simulink model "test_direct"  (R2024a)
settings: Solver=VariableStepAuto  StartTime=0.0  StopTime=40  RelTol=1e-3
libraries: neural x733, simulink x4
(part 20 of 35)

== system test_direct/Function Fitting Neural Network3/Layer 4/Delays 1 ==
  "p{4}" : Inport  PortDimensions=20
      mask Display: e = 0.06;c1 = [120 230 180]/255;c2 = ([120 230 180]+0)/(256+128);c3 = ([120 230 180]+128)/(256+128);patch([0 1 1 0],[0 0 1 1],c1);patch([0 1 1 1-e 1-e 0+e],[0 0 1 1-e 0+e 0+e],c2);patch([0 0 1 1-e 0+e 0+e],[0 1 1 1-e 1-e 0+e],c3);plot([0 1 1 0 0],[0 0 1 1 0]);
  mux : Mux  Inputs=1
      mask Display: e = 0.06;c1 = [120 150 230]/255;c2 = ([120 150 230]+0)/383;c3 = ([120 150 230]+128)/383;patch([0 1 1 0],[0 0 1 1],c1);patch([0 1 1 1-e 1-e 0+e],[0 0 1 1-e 0+e 0+e],c2);patch([0 0 1 1-e 0+e 0+e],[0 1 1 1-e 1-e 0+e],c3);plot([0 1 1 0 0],[0 0 1 1 0]);disp('Mux')
  "pd{4,3}" : Outport
      mask Display: e = 0.06;c1 = [120 230 180]/255;c2 = ([120 230 180]+0)/(256+128);c3 = ([120 230 180]+128)/(256+128);patch([0 1 1 0],[0 0 1 1],c1);patch([0 1 1 1-e 1-e 0+e],[0 0 1 1-e 0+e 0+e],c2);patch([0 0 1 1-e 0+e 0+e],[0 1 1 1-e 1-e 0+e],c3);plot([0 1 1 0 0],[0 0 1 1 0]);
  wires:
  "p{4}"/1 -> mux/1
  mux/1 -> "pd{4,3}"/1

== system test_direct/Function Fitting Neural Network3/Layer 4/LW{4,3} ==
  "ad{4,3}" : Inport  PortDimensions=20
      mask Display: e = 0.06;c1 = [120 230 180]/255;c2 = ([120 230 180]+0)/(256+128);c3 = ([120 230 180]+128)/(256+128);patch([0 1 1 0],[0 0 1 1],c1);patch([0 1 1 1-e 1-e 0+e],[0 0 1 1-e 0+e 0+e],c2);patch([0 0 1 1-e 0+e 0+e],[0 1 1 1-e 1-e 0+e],c3);plot([0 1 1 0 0],[0 0 1 1 0]);
  "IW{4,3}(1,:)'" : Constant  Value=[-0.48686646195795912905879276877385564148426055908203125;-0.039175733463625579677813703938227263279259204864501953125;-0.054262605722279790010365019270466291345655918121337890625;-0.0940799827120739617924982667318545281887054443359375;0.368204999001782551371064755585393868386745452880859375;-0.060856578835075413047572823188602342270314693450927734375;-0.016079589379415247518689824346438399516046047210693359375;-0.5573541309042620017777380780898965895175933837890625;-0.410950220679517475019792982493527233600616455078125;-0.456090081196367957971915529924444854259490966796875;-0.086733219532944494378767785747186280786991119384765625;-0.442442468295296709168695770131307654082775115966796875;0.181816513039095795090105411873082630336284637451171875;0.324817807046969997397667384575470350682735443115234375;0.0251481921723479238950371694727436988614499568939208984375;-0.233647632030154317472891989382333122193813323974609375;0.47822246659309808336502101155929267406463623046875;-0.281298981443819762215952096084947697818279266357421875;-0.342982629902267077692812335953931324183940887451171875;0.111229079439892408753820518541033379733562469482421875]
      mask Display: e = 0.06;c1 = [120 150 230]/255;c2 = ([120 150 230]+0)/383;c3 = ([120 150 230]+128)/383;patch([0 1 1 0],[0 0 1 1],c1);patch([0 1 1 1-e 1-e 0+e],[0 0 1 1-e 0+e 0+e],c2);patch([0 0 1 1-e 0+e 0+e],[0 1 1 1-e 1-e 0+e],c3);plot([0 1 1 0 0],[0 0 1 1 0]);disp('weights');
  "IW{4,3}(10,:)'" : Constant  Value=[0.1322689043770106653852280942373909056186676025390625;0.58032543371156875000593799995840527117252349853515625;0.2470434001325927386716330147464759647846221923828125;0.381612023463914373788696821065968833863735198974609375;0.46510415946604710679679328677593730390071868896484375;0.36918358843860288320826157359988428652286529541015625;0.10829240045879288956154340439752559177577495574951171875;0.438447426649319738078958152982522733509540557861328125;-0.475651030999239221586094572558067739009857177734375;0.5174868322376242613103158873855136334896087646484375;0.46252837137097035924426791098085232079029083251953125;0.351788445832689256054237603166257031261920928955078125;0.2169410354624995151961996953104971908032894134521484375;-0.003875396627683679907916403095669011236168444156646728515625;0.04911082881832169733105075692947139032185077667236328125;0.052739315397494108961229386522973072715103626251220703125;-0.05480510469211240243136984418015344999730587005615234375;-0.53198177995099904524778366976534016430377960205078125;-0.10334524086508810325479856828678748570382595062255859375;0.375453827597210965105745117398328147828578948974609375]
      mask Display: e = 0.06;c1 = [120 150 230]/255;c2 = ([120 150 230]+0)/383;c3 = ([120 150 230]+128)/383;patch([0 1 1 0],[0 0 1 1],c1);patch([0 1 1 1-e 1-e 0+e],[0 0 1 1-e 0+e 0+e],c2);patch([0 0 1 1-e 0+e 0+e],[0 1 1 1-e 1-e 0+e],c3);plot([0 1 1 0 0],[0 0 1 1 0]);disp('weights');
  "IW{4,3}(2,:)'" : Constant  Value=[0.394185608854831726066691999221802689135074615478515625;-0.73688134269214800031733147989143617451190948486328125;0.07487875784436172355018612734056659974157810211181640625;0.422127005558921297723173893245984800159931182861328125;-0.1848428640511568799009722852133563719689846038818359375;0.093106201221737350248730535895447246730327606201171875;-0.639864400764405427679548665764741599559783935546875;-0.45328319723072063585078694814001210033893585205078125;0.58552337302374535266125121779623441398143768310546875;0.1926483079783262442052915730528184212744235992431640625;-0.60409923873878768052492205242742784321308135986328125;0.468018274699262659677145848036161623895168304443359375;-0.8511680335689548737576615167199634015560150146484375;0.024315010267243752917210031228023581206798553466796875;0.224700621110978493444321202332503162324428558349609375;-0.0016341048010425356269703645040181072545237839221954345703125;0.020521423701335757272534721096235443837940692901611328125;-0.214964210107415232275940297768102027475833892822265625;0.48652592408502892684651897070580162107944488525390625;-0.50226604360123972004004144764621742069721221923828125]
      mask Display: e = 0.06;c1 = [120 150 230]/255;c2 = ([120 150 230]+0)/383;c3 = ([120 150 230]+128)/383;patch([0 1 1 0],[0 0 1 1],c1);patch([0 1 1 1-e 1-e 0+e],[0 0 1 1-e 0+e 0+e],c2);patch([0 0 1 1-e 0+e 0+e],[0 1 1 1-e 1-e 0+e],c3);plot([0 1 1 0 0],[0 0 1 1 0]);disp('weights');
  "IW{4,3}(3,:)'" : Constant  Value=[-0.2491793519076358764952061619624146260321140289306640625;0.2423952947801428503549203696820768527686595916748046875;-0.446054257266220999245120992782176472246646881103515625;-0.54592514430021055193975598740507848560810089111328125;0.339034794585557353041593842135625891387462615966796875;0.1746683376047669933317507684478187002241611480712890625;-0.352707257123562489820045584565377794206142425537109375;0.045936039691991246980418139855828485451638698577880859375;-0.1638667128451297971825084687225171364843845367431640625;0.250704205658886014607134029574808664619922637939453125;-0.294664529227201210659359276178292930126190185546875;-0.42733283149903389386281560291536152362823486328125;0.2269107231504099153607256766917998902499675750732421875;0.57311441583918953934784212833619676530361175537109375;-0.30882524085834373028802701810491271317005157470703125;0.42145837800391727778759332068148069083690643310546875;0.01697039272420101940763714765125769190490245819091796875;0.33169200899486928069137547936406917870044708251953125;-0.493372721243436063165432869936921633780002593994140625;0.6407201682409671139595275235478766262531280517578125]
      mask Display: e = 0.06;c1 = [120 150 230]/255;c2 = ([120 150 230]+0)/383;c3 = ([120 150 230]+128)/383;patch([0 1 1 0],[0 0 1 1],c1);patch([0 1 1 1-e 1-e 0+e],[0 0 1 1-e 0+e 0+e],c2);patch([0 0 1 1-e 0+e 0+e],[0 1 1 1-e 1-e 0+e],c3);plot([0 1 1 0 0],[0 0 1 1 0]);disp('weights');
  "IW{4,3}(4,:)'" : Constant  Value=[-0.185259915495485427694433155920705758035182952880859375;-0.0602096723483524220998930331916199065744876861572265625;0.005160964867985998703880934357357546105049550533294677734375;-0.28022125227828265092711035322281531989574432373046875;-0.260470767970210126396324312736396677792072296142578125;-0.061202911858095128405654605785457533784210681915283203125;-0.1114271602009062334115441217363695614039897918701171875;0.65705660638789586958097288516000844538211822509765625;0.0274548355082907501178990372636690153740346431732177734375;0.0196237861339672824134705564347314066253602504730224609375;0.181669946716588370794198681323905475437641143798828125;-0.337641594933245914322839098531403578817844390869140625;-0.1374064240998444652586130132476682774722576141357421875;-0.1853221345637752204282833190518431365489959716796875;-0.65902271493018016457199337310157716274261474609375;-0.1235825644534767897564364602658315561711788177490234375;-0.2164996901666107198547450707337702624499797821044921875;0.465730287211794602431069733938784338533878326416015625;-0.0225226151377865453639959270049075712449848651885986328125;0.453007245753051457359816822645370848476886749267578125]
      mask Display: e = 0.06;c1 = [120 150 230]/255;c2 = ([120 150 230]+0)/383;c3 = ([120 150 230]+128)/383;patch([0 1 1 0],[0 0 1 1],c1);patch([0 1 1 1-e 1-e 0+e],[0 0 1 1-e 0+e 0+e],c2);patch([0 0 1 1-e 0+e 0+e],[0 1 1 1-e 1-e 0+e],c3);plot([0 1 1 0 0],[0 0 1 1 0]);disp('weights');
  "IW{4,3}(5,:)'" : Constant  Value=[-0.428439923209114059687863118597306311130523681640625;-0.479089500144313007456986497345496900379657745361328125;-0.475435563334728195084011304061277769505977630615234375;0.28555488193449340972307481933967210352420806884765625;-0.0671512868641155058480052275626803748309612274169921875;-0.103174105025102991195495860665687359869480133056640625;0.1779694070506021574828992015682160854339599609375;-0.4165875142106241213468820205889642238616943359375;0.11253138387435483724896556623207288794219493865966796875;-0.414639990588654028247361793546588160097599029541015625;0.5106068345219061388462478134897537529468536376953125;-0.442561665969515571905645856531918980181217193603515625;0.1283178924385620367498717087073600850999355316162109375;0.288453901604045104267726173929986543953418731689453125;0.4438188348713214548268979342537932097911834716796875;0.31938958024108232702786835943697951734066009521484375;-0.08115556966456148602073739084517001174390316009521484375;0.293674793410225898337984062891337089240550994873046875;0.2448754137198137226238969788028043694794178009033203125;0.5552223354759082685205839879927225410938262939453125]
      mask Display: e = 0.06;c1 = [120 150 230]/255;c2 = ([120 150 230]+0)/383;c3 = ([120 150 230]+128)/383;patch([0 1 1 0],[0 0 1 1],c1);patch([0 1 1 1-e 1-e 0+e],[0 0 1 1-e 0+e 0+e],c2);patch([0 0 1 1-e 0+e 0+e],[0 1 1 1-e 1-e 0+e],c3);plot([0 1 1 0 0],[0 0 1 1 0]);disp('weights');
  "IW{4,3}(6,:)'" : Constant  Value=[-0.49335970568954834458708091915468685328960418701171875;0.627254380166531344542590886703692376613616943359375;-0.42687565884003342286945326122804544866085052490234375;-0.8096754077238739188970839677494950592517852783203125;-0.57129515370796724038626734909485094249248504638671875;0.5820748227951784148359593018540181219577789306640625;0.85048395815353872162489778929739259183406829833984375;0.08899992698425469861422953954388503916561603546142578125;-1.08570552066859793427511249319650232791900634765625;0.462303758497051131559629766343277879059314727783203125;-0.903259753431511658305907985777594149112701416015625;0.10726998787899404141921166910833562724292278289794921875;0.465031374451071066733476300214533694088459014892578125;-0.45929324220655354249487345441593788564205169677734375;-0.56223262128137729831678370828740298748016357421875;0.339090944158511431449909423463395796716213226318359375;-0.11761342441935905556160690821343450807034969329833984375;-0.37686279254677323979905168016557581722736358642578125;0.04121241225336517988164786174820619635283946990966796875;-0.2042736093037561817542524522650637663900852203369140625]
      mask Display: e = 0.06;c1 = [120 150 230]/255;c2 = ([120 150 230]+0)/383;c3 = ([120 150 230]+128)/383;patch([0 1 1 0],[0 0 1 1],c1);patch([0 1 1 1-e 1-e 0+e],[0 0 1 1-e 0+e 0+e],c2);patch([0 0 1 1-e 0+e 0+e],[0 1 1 1-e 1-e 0+e],c3);plot([0 1 1 0 0],[0 0 1 1 0]);disp('weights');
  "IW{4,3}(7,:)'" : Constant  Value=[-0.06537952429101571982794638415725785307586193084716796875;0.0686118153796015095569060804336913861334323883056640625;-0.2105712354158649490809551707570790313184261322021484375;0.05224571883096605640073306631165905855596065521240234375;0.007546513790575325175691290269242017529904842376708984375;0.083163865197247666127822185444529168307781219482421875;0.27287292560545661768145464520785026252269744873046875;0.438194139001469362693086395665886811912059783935546875;-0.034300814531695124343091407581596286036074161529541015625;0.51963615226882031716826304545975290238857269287109375;0.6487591374666166199602912456612102687358856201171875;-0.463435073667250396756145391918835230171680450439453125;0.002905004743866214378389400962987565435469150543212890625;0.73084099932672652588649953031563200056552886962890625;-0.4272768910794726426871648072847165167331695556640625;0.3072026547358976955592879676260054111480712890625;-0.307773827519164100419146734566311351954936981201171875;-0.283230198793040177651647582024452276527881622314453125;-0.1218488722444253935517366471685818396508693695068359375;-0.00267663631928003430127116502035278244875371456146240234375]
      mask Display: e = 0.06;c1 = [120 150 230]/255;c2 = ([120 150 230]+0)/383;c3 = ([120 150 230]+128)/383;patch([0 1 1 0],[0 0 1 1],c1);patch([0 1 1 1-e 1-e 0+e],[0 0 1 1-e 0+e 0+e],c2);patch([0 0 1 1-e 0+e 0+e],[0 1 1 1-e 1-e 0+e],c3);plot([0 1 1 0 0],[0 0 1 1 0]);disp('weights');
  "IW{4,3}(8,:)'" : Constant  Value=[0.5905066251936845755921012823819182813167572021484375;-0.30329863794689615463795462346752174198627471923828125;-0.09760906261871506173211088253083289600908756256103515625;-0.2429638526781317808822535653234808705747127532958984375;0.3234179069280116447515638355980627238750457763671875;-0.42333294766016471566416612404282204806804656982421875;0.3236234153818726699824992465437389910221099853515625;0.441875449522532603996438638205290772020816802978515625;0.5068013555949091308860943172476254403591156005859375;-0.1972272324421973921371176174943684600293636322021484375;0.0480240103525966521846868317879852838814258575439453125;0.444141970587676127024678862653672695159912109375;-0.2197429979112982822986310793567099608480930328369140625;-0.6816575021358606267796176325646229088306427001953125;-0.7021329850213240408862702679471112787723541259765625;-0.411567756854281541212259298845310695469379425048828125;-0.1317867912264614194128853341680951416492462158203125;-0.462287294868110543166750403543119318783283233642578125;0.34924752008150428128629982893471606075763702392578125;0.10496481903143962954860768377329804934561252593994140625]
      mask Display: e = 0.06;c1 = [120 150 230]/255;c2 = ([120 150 230]+0)/383;c3 = ([120 150 230]+128)/383;patch([0 1 1 0],[0 0 1 1],c1);patch([0 1 1 1-e 1-e 0+e],[0 0 1 1-e 0+e 0+e],c2);patch([0 0 1 1-e 0+e 0+e],[0 1 1 1-e 1-e 0+e],c3);plot([0 1 1 0 0],[0 0 1 1 0]);disp('weights');
  "IW{4,3}(9,:)'" : Constant  Value=[0.43056348001155819726903928312822245061397552490234375;0.00111634494525898330004320957442587314289994537830352783203125;-0.528135750842535944826749982894398272037506103515625;-0.307078785122185227152158404351212084293365478515625;-0.03333149626931240783189736021085991524159908294677734375;-0.1371153453742978423068876736579113639891147613525390625;-0.06662096833313123356301588273709057830274105072021484375;0.452089390549744785108288169794832356274127960205078125;0.67958178908102506721178315274300985038280487060546875;-0.362801795077034749947841874018195085227489471435546875;0.339735254339901426856584976121666841208934783935546875;-0.4909941905178099030848670736304484307765960693359375;0.330655951855933827321365470197633840143680572509765625;-0.339969929699753758978175710581126622855663299560546875;-0.0965979905593430110410935185427661053836345672607421875;0.1254839413117765645200307744744350202381610870361328125;0.35972773789546763634206172355334274470806121826171875;-0.2147232346809808678500530731980688869953155517578125;0.48694385960235730959055899802478961646556854248046875;0.172732370055611317294363971086568199098110198974609375]
      mask Display: e = 0.06;c1 = [120 150 230]/255;c2 = ([120 150 230]+0)/383;c3 = ([120 150 230]+128)/383;patch([0 1 1 0],[0 0 1 1],c1);patch([0 1 1 1-e 1-e 0+e],[0 0 1 1-e 0+e 0+e],c2);patch([0 0 1 1-e 0+e 0+e],[0 1 1 1-e 1-e 0+e],c3);plot([0 1 1 0 0],[0 0 1 1 0]);disp('weights');
  Mux : Mux  Inputs=10
      mask Display: e = 0.06;c1 = [120 150 230]/255;c2 = ([120 150 230]+0)/383;c3 = ([120 150 230]+128)/383;patch([0 1 1 0],[0 0 1 1],c1);patch([0 1 1 1-e 1-e 0+e],[0 0 1 1-e 0+e 0+e],c2);patch([0 0 1 1-e 0+e 0+e],[0 1 1 1-e 1-e 0+e],c3);plot([0 1 1 0 0],[0 0 1 1 0]);disp('Mux');
  dotprod{1..10} (10 alike) : neural/Weight Functions/dotprod
  "lz{4,3}" : Outport
      mask Display: e = 0.06;c1 = [120 230 180]/255;c2 = ([120 230 180]+0)/(256+128);c3 = ([120 230 180]+128)/(256+128);patch([0 1 1 0],[0 0 1 1],c1);patch([0 1 1 1-e 1-e 0+e],[0 0 1 1-e 0+e 0+e],c2);patch([0 0 1 1-e 0+e 0+e],[0 1 1 1-e 1-e 0+e],c3);plot([0 1 1 0 0],[0 0 1 1 0]);
  wires:
  "IW{4,3}(1,:)'"/1 -> dotprod1/1
  "ad{4,3}"/1 -> dotprod1/2, dotprod2/2, dotprod3/2, dotprod4/2, dotprod5/2, dotprod6/2, dotprod7/2, dotprod8/2, dotprod9/2, dotprod10/2
  dotprod1/1 -> Mux/1
  "IW{4,3}(2,:)'"/1 -> dotprod2/1
  dotprod2/1 -> Mux/2
  "IW{4,3}(3,:)'"/1 -> dotprod3/1
  dotprod3/1 -> Mux/3
  "IW{4,3}(4,:)'"/1 -> dotprod4/1
  dotprod4/1 -> Mux/4
  "IW{4,3}(5,:)'"/1 -> dotprod5/1
  dotprod5/1 -> Mux/5
  "IW{4,3}(6,:)'"/1 -> dotprod6/1
  dotprod6/1 -> Mux/6
  "IW{4,3}(7,:)'"/1 -> dotprod7/1
  dotprod7/1 -> Mux/7
  "IW{4,3}(8,:)'"/1 -> dotprod8/1
  dotprod8/1 -> Mux/8
  "IW{4,3}(9,:)'"/1 -> dotprod9/1
  dotprod9/1 -> Mux/9
  "IW{4,3}(10,:)'"/1 -> dotprod10/1
  dotprod10/1 -> Mux/10
  Mux/1 -> "lz{4,3}"/1

== system test_direct/Function Fitting Neural Network3/Layer 5/Delays 1 ==
  "p{5}" : Inport  PortDimensions=10
      mask Display: e = 0.06;c1 = [120 230 180]/255;c2 = ([120 230 180]+0)/(256+128);c3 = ([120 230 180]+128)/(256+128);patch([0 1 1 0],[0 0 1 1],c1);patch([0 1 1 1-e 1-e 0+e],[0 0 1 1-e 0+e 0+e],c2);patch([0 0 1 1-e 0+e 0+e],[0 1 1 1-e 1-e 0+e],c3);plot([0 1 1 0 0],[0 0 1 1 0]);
  mux : Mux  Inputs=1
      mask Display: e = 0.06;c1 = [120 150 230]/255;c2 = ([120 150 230]+0)/383;c3 = ([120 150 230]+128)/383;patch([0 1 1 0],[0 0 1 1],c1);patch([0 1 1 1-e 1-e 0+e],[0 0 1 1-e 0+e 0+e],c2);patch([0 0 1 1-e 0+e 0+e],[0 1 1 1-e 1-e 0+e],c3);plot([0 1 1 0 0],[0 0 1 1 0]);disp('Mux')
  "pd{5,4}" : Outport
      mask Display: e = 0.06;c1 = [120 230 180]/255;c2 = ([120 230 180]+0)/(256+128);c3 = ([120 230 180]+128)/(256+128);patch([0 1 1 0],[0 0 1 1],c1);patch([0 1 1 1-e 1-e 0+e],[0 0 1 1-e 0+e 0+e],c2);patch([0 0 1 1-e 0+e 0+e],[0 1 1 1-e 1-e 0+e],c3);plot([0 1 1 0 0],[0 0 1 1 0]);
  wires:
  "p{5}"/1 -> mux/1
  mux/1 -> "pd{5,4}"/1

== system test_direct/Function Fitting Neural Network3/Layer 5/LW{5,4} ==
  "ad{5,4}" : Inport  PortDimensions=10
      mask Display: e = 0.06;c1 = [120 230 180]/255;c2 = ([120 230 180]+0)/(256+128);c3 = ([120 230 180]+128)/(256+128);patch([0 1 1 0],[0 0 1 1],c1);patch([0 1 1 1-e 1-e 0+e],[0 0 1 1-e 0+e 0+e],c2);patch([0 0 1 1-e 0+e 0+e],[0 1 1 1-e 1-e 0+e],c3);plot([0 1 1 0 0],[0 0 1 1 0]);
  "IW{5,4}(1,:)'" : Constant  Value=[1.0708531371956653277521809286554343998432159423828125;1.2177692914654476563640628228313289582729339599609375;-0.77496673536313653851692606622236780822277069091796875;-1.0430073552631797806355962165980599820613861083984375;0.54831452182435735931420595079544000327587127685546875;-0.395600858983294167980915290172561071813106536865234375;-0.109788596365533563936622840628842823207378387451171875;0.213357739162486570450028011691756546497344970703125;-0.28566082510756130030671329222968779504299163818359375;0.09187921716738935151713718596511171199381351470947265625]
      mask Display: e = 0.06;c1 = [120 150 230]/255;c2 = ([120 150 230]+0)/383;c3 = ([120 150 230]+128)/383;patch([0 1 1 0],[0 0 1 1],c1);patch([0 1 1 1-e 1-e 0+e],[0 0 1 1-e 0+e 0+e],c2);patch([0 0 1 1-e 0+e 0+e],[0 1 1 1-e 1-e 0+e],c3);plot([0 1 1 0 0],[0 0 1 1 0]);disp('weights');
  "IW{5,4}(2,:)'" : Constant  Value=[1.0181111840726746464724783436395227909088134765625;-1.0581252028500636175323279530857689678668975830078125;0.037743756557340878143858020621337345801293849945068359375;-0.190503982491262935372589026883360929787158966064453125;0.83413814930360918875607012523687444627285003662109375;1.540630667106828610712909721769392490386962890625;-0.546343038711933015605382024659775197505950927734375;1.046855860728096221379246344440616667270660400390625;0.0195656728667780409336440783363286755047738552093505859375;-0.3293391962601022182610677191405557096004486083984375]
      mask Display: e = 0.06;c1 = [120 150 230]/255;c2 = ([120 150 230]+0)/383;c3 = ([120 150 230]+128)/383;patch([0 1 1 0],[0 0 1 1],c1);patch([0 1 1 1-e 1-e 0+e],[0 0 1 1-e 0+e 0+e],c2);patch([0 0 1 1-e 0+e 0+e],[0 1 1 1-e 1-e 0+e],c3);plot([0 1 1 0 0],[0 0 1 1 0]);disp('weights');
  Mux : Mux  Inputs=2
      mask Display: e = 0.06;c1 = [120 150 230]/255;c2 = ([120 150 230]+0)/383;c3 = ([120 150 230]+128)/383;patch([0 1 1 0],[0 0 1 1],c1);patch([0 1 1 1-e 1-e 0+e],[0 0 1 1-e 0+e 0+e],c2);patch([0 0 1 1-e 0+e 0+e],[0 1 1 1-e 1-e 0+e],c3);plot([0 1 1 0 0],[0 0 1 1 0]);disp('Mux');
  dotprod1 : neural/Weight Functions/dotprod
  dotprod2 : neural/Weight Functions/dotprod
  "lz{5,4}" : Outport
      mask Display: e = 0.06;c1 = [120 230 180]/255;c2 = ([120 230 180]+0)/(256+128);c3 = ([120 230 180]+128)/(256+128);patch([0 1 1 0],[0 0 1 1],c1);patch([0 1 1 1-e 1-e 0+e],[0 0 1 1-e 0+e 0+e],c2);patch([0 0 1 1-e 0+e 0+e],[0 1 1 1-e 1-e 0+e],c3);plot([0 1 1 0 0],[0 0 1 1 0]);
  wires:
  "IW{5,4}(1,:)'"/1 -> dotprod1/1
  "ad{5,4}"/1 -> dotprod1/2, dotprod2/2
  dotprod1/1 -> Mux/1
  "IW{5,4}(2,:)'"/1 -> dotprod2/1
  dotprod2/1 -> Mux/2
  Mux/1 -> "lz{5,4}"/1

== system test_direct/Function Fitting Neural Network4/Layer 1/Delays 1 ==
  "p{1}" : Inport  PortDimensions=8
      mask Display: e = 0.06;c1 = [120 230 180]/255;c2 = ([120 230 180]+0)/(256+128);c3 = ([120 230 180]+128)/(256+128);patch([0 1 1 0],[0 0 1 1],c1);patch([0 1 1 1-e 1-e 0+e],[0 0 1 1-e 0+e 0+e],c2);patch([0 0 1 1-e 0+e 0+e],[0 1 1 1-e 1-e 0+e],c3);plot([0 1 1 0 0],[0 0 1 1 0]);
  mux : Mux  Inputs=1
      mask Display: e = 0.06;c1 = [120 150 230]/255;c2 = ([120 150 230]+0)/383;c3 = ([120 150 230]+128)/383;patch([0 1 1 0],[0 0 1 1],c1);patch([0 1 1 1-e 1-e 0+e],[0 0 1 1-e 0+e 0+e],c2);patch([0 0 1 1-e 0+e 0+e],[0 1 1 1-e 1-e 0+e],c3);plot([0 1 1 0 0],[0 0 1 1 0]);disp('Mux')
  "pd{1,1}" : Outport
      mask Display: e = 0.06;c1 = [120 230 180]/255;c2 = ([120 230 180]+0)/(256+128);c3 = ([120 230 180]+128)/(256+128);patch([0 1 1 0],[0 0 1 1],c1);patch([0 1 1 1-e 1-e 0+e],[0 0 1 1-e 0+e 0+e],c2);patch([0 0 1 1-e 0+e 0+e],[0 1 1 1-e 1-e 0+e],c3);plot([0 1 1 0 0],[0 0 1 1 0]);
  wires:
  "p{1}"/1 -> mux/1
  mux/1 -> "pd{1,1}"/1

== system test_direct/Function Fitting Neural Network4/Layer 1/IW{1,1} ==
  "pd{1,1}" : Inport  PortDimensions=8
      mask Display: e = 0.06;c1 = [120 230 180]/255;c2 = ([120 230 180]+0)/(256+128);c3 = ([120 230 180]+128)/(256+128);patch([0 1 1 0],[0 0 1 1],c1);patch([0 1 1 1-e 1-e 0+e],[0 0 1 1-e 0+e 0+e],c2);patch([0 0 1 1-e 0+e 0+e],[0 1 1 1-e 1-e 0+e],c3);plot([0 1 1 0 0],[0 0 1 1 0]);
  "IW{1,1}(1,:)'" : Constant  Value=[-0.06625151497961288826754611136493622325360774993896484375;0.09601682548573871323061013072219793684780597686767578125;-0.60795817852282940663144472637213766574859619140625;0.32346487533894763277686479341355152428150177001953125;-0.417565763028574454818198091743397526443004608154296875;-1.2591612239835876518867507911636494100093841552734375;-0.0166700018866756151381114392506788135506212711334228515625;-0.99469795689098761126700765089481137692928314208984375]
      mask Display: e = 0.06;c1 = [120 150 230]/255;c2 = ([120 150 230]+0)/383;c3 = ([120 150 230]+128)/383;patch([0 1 1 0],[0 0 1 1],c1);patch([0 1 1 1-e 1-e 0+e],[0 0 1 1-e 0+e 0+e],c2);patch([0 0 1 1-e 0+e 0+e],[0 1 1 1-e 1-e 0+e],c3);plot([0 1 1 0 0],[0 0 1 1 0]);disp('Weights');
  "IW{1,1}(10,:)'" : Constant  Value=[-0.07805198563980701720321775383126805536448955535888671875;0.132721065130629700679065763324615545570850372314453125;-0.61744434245293489116335194921703077852725982666015625;0.388935332600696181959420982821029610931873321533203125;0.153285063860497727805665135747403837740421295166015625;0.50930623689561549394255735023762099444866180419921875;0.53845382130426389100108508500852622091770172119140625;0.497782563507082276288429056876339018344879150390625]
      mask Display: e = 0.06;c1 = [120 150 230]/255;c2 = ([120 150 230]+0)/383;c3 = ([120 150 230]+128)/383;patch([0 1 1 0],[0 0 1 1],c1);patch([0 1 1 1-e 1-e 0+e],[0 0 1 1-e 0+e 0+e],c2);patch([0 0 1 1-e 0+e 0+e],[0 1 1 1-e 1-e 0+e],c3);plot([0 1 1 0 0],[0 0 1 1 0]);disp('Weights');
  "IW{1,1}(11,:)'" : Constant  Value=[0.04918441610870837032987168413455947302281856536865234375;-0.04159552238430817838743536185575067065656185150146484375;0.12327812348590654056845750119464355520904064178466796875;0.06319189768471338009003801516882958821952342987060546875;0.056797211991516181883721259282538085244596004486083984375;-2.039553404596769592416194427642039954662322998046875;0.039085160146814422466032823422210640273988246917724609375;0.7273537078235470243470217610592953860759735107421875]
      mask Display: e = 0.06;c1 = [120 150 230]/255;c2 = ([120 150 230]+0)/383;c3 = ([120 150 230]+128)/383;patch([0 1 1 0],[0 0 1 1],c1);patch([0 1 1 1-e 1-e 0+e],[0 0 1 1-e 0+e 0+e],c2);patch([0 0 1 1-e 0+e 0+e],[0 1 1 1-e 1-e 0+e],c3);plot([0 1 1 0 0],[0 0 1 1 0]);disp('Weights');
  "IW{1,1}(12,:)'" : Constant  Value=[-0.00167045469516673259109673654876360160415060818195343017578125;0.01347407452638137159706133161307661794126033782958984375;-0.1851645838153682943616473721704096533358097076416015625;-0.11655323356809062229633155993724358268082141876220703125;-0.62722879354085936398632838972844183444976806640625;-1.1853717592089576537972561709466390311717987060546875;0.95522238224009192730790118730510585010051727294921875;0.431675565915472347899850547037203796207904815673828125]
      mask Display: e = 0.06;c1 = [120 150 230]/255;c2 = ([120 150 230]+0)/383;c3 = ([120 150 230]+128)/383;patch([0 1 1 0],[0 0 1 1],c1);patch([0 1 1 1-e 1-e 0+e],[0 0 1 1-e 0+e 0+e],c2);patch([0 0 1 1-e 0+e 0+e],[0 1 1 1-e 1-e 0+e],c3);plot([0 1 1 0 0],[0 0 1 1 0]);disp('Weights');
  "IW{1,1}(13,:)'" : Constant  Value=[0.039281083063148487799498553840749082155525684356689453125;-0.0064241656681929791561369569308226346038281917572021484375;-0.211170003365020397811946395449922420084476470947265625;0.10621998061268729529604826211652834899723529815673828125;0.8272839260666058347482021417818032205104827880859375;-0.01424818209783466731177536956920448574237525463104248046875;-1.27198045641837875763258125516586005687713623046875;-0.4679124231279334633626376671600155532360076904296875]
      mask Display: e = 0.06;c1 = [120 150 230]/255;c2 = ([120 150 230]+0)/383;c3 = ([120 150 230]+128)/383;patch([0 1 1 0],[0 0 1 1],c1);patch([0 1 1 1-e 1-e 0+e],[0 0 1 1-e 0+e 0+e],c2);patch([0 0 1 1-e 0+e 0+e],[0 1 1 1-e 1-e 0+e],c3);plot([0 1 1 0 0],[0 0 1 1 0]);disp('Weights');
  "IW{1,1}(14,:)'" : Constant  Value=[-0.0169495841255620262322256763809491530992090702056884765625;0.01062986111865275341836767353242976241745054721832275390625;1.30927265313393714762923991656862199306488037109375;0.63133840280491126950579428012133575975894927978515625;-0.96762180382265527978091768090962432324886322021484375;0.1618197698033403408857111571705900132656097412109375;0.86217582271051107500881016676430590450763702392578125;0.339944606698661277999207186439889483153820037841796875]
      mask Display: e = 0.06;c1 = [120 150 230]/255;c2 = ([120 150 230]+0)/383;c3 = ([120 150 230]+128)/383;patch([0 1 1 0],[0 0 1 1],c1);patch([0 1 1 1-e 1-e 0+e],[0 0 1 1-e 0+e 0+e],c2);patch([0 0 1 1-e 0+e 0+e],[0 1 1 1-e 1-e 0+e],c3);plot([0 1 1 0 0],[0 0 1 1 0]);disp('Weights');
  "IW{1,1}(15,:)'" : Constant  Value=[0.0373943282553832745396249492841889150440692901611328125;-0.050913543636903757505507428504643030464649200439453125;0.058094347573448119892436380951039609499275684356689453125;0.03971616806807866384421146221939125098288059234619140625;-0.2137823796082287952646794337852043099701404571533203125;0.2076334074508816851523107516186428256332874298095703125;-0.1636610146309179503187891668858355842530727386474609375;-1.476979632139391096501412903307937085628509521484375]
      mask Display: e = 0.06;c1 = [120 150 230]/255;c2 = ([120 150 230]+0)/383;c3 = ([120 150 230]+128)/383;patch([0 1 1 0],[0 0 1 1],c1);patch([0 1 1 1-e 1-e 0+e],[0 0 1 1-e 0+e 0+e],c2);patch([0 0 1 1-e 0+e 0+e],[0 1 1 1-e 1-e 0+e],c3);plot([0 1 1 0 0],[0 0 1 1 0]);disp('Weights');
  "IW{1,1}(16,:)'" : Constant  Value=[0.10879873244421413291949107815526076592504978179931640625;-0.10022134176543344430410087397831375710666179656982421875;0.144544047383925511329749724609428085386753082275390625;-0.165210772886099588330210963249555788934230804443359375;0.193923316401156842214703601712244562804698944091796875;0.259818504779267211990401165166986174881458282470703125;0.489322251805624885978573956890613771975040435791015625;-1.076272524477527969821721853804774582386016845703125]
      mask Display: e = 0.06;c1 = [120 150 230]/255;c2 = ([120 150 230]+0)/383;c3 = ([120 150 230]+128)/383;patch([0 1 1 0],[0 0 1 1],c1);patch([0 1 1 1-e 1-e 0+e],[0 0 1 1-e 0+e 0+e],c2);patch([0 0 1 1-e 0+e 0+e],[0 1 1 1-e 1-e 0+e],c3);plot([0 1 1 0 0],[0 0 1 1 0]);disp('Weights');
  "IW{1,1}(17,:)'" : Constant  Value=[0.038510554429168834811303412379857036285102367401123046875;-0.0404876974188733418369423588956124149262905120849609375;-0.46506761858084322280859623788273893296718597412109375;-0.36389906569615682041529680645908229053020477294921875;-0.824413710546632483300300009432248771190643310546875;0.355521399529579895659736621382762677967548370361328125;0.4848339535763752650154856382869184017181396484375;-1.1917727827283621788723166901036165654659271240234375]
      mask Display: e = 0.06;c1 = [120 150 230]/255;c2 = ([120 150 230]+0)/383;c3 = ([120 150 230]+128)/383;patch([0 1 1 0],[0 0 1 1],c1);patch([0 1 1 1-e 1-e 0+e],[0 0 1 1-e 0+e 0+e],c2);patch([0 0 1 1-e 0+e 0+e],[0 1 1 1-e 1-e 0+e],c3);plot([0 1 1 0 0],[0 0 1 1 0]);disp('Weights');
  "IW{1,1}(18,:)'" : Constant  Value=[0.60227918242615363642045167580363340675830841064453125;-0.7151315300296705590454848788795061409473419189453125;0.492170888404110218328213477434474043548107147216796875;-0.41266629077125893676480927751981653273105621337890625;0.060275798823175567864307566878778743557631969451904296875;0.06632476508515561253176429090672172605991363525390625;0.468340613243486580952179565429105423390865325927734375;-0.75850147031254433471758602536283433437347412109375]
      mask Display: e = 0.06;c1 = [120 150 230]/255;c2 = ([120 150 230]+0)/383;c3 = ([120 150 230]+128)/383;patch([0 1 1 0],[0 0 1 1],c1);patch([0 1 1 1-e 1-e 0+e],[0 0 1 1-e 0+e 0+e],c2);patch([0 0 1 1-e 0+e 0+e],[0 1 1 1-e 1-e 0+e],c3);plot([0 1 1 0 0],[0 0 1 1 0]);disp('Weights');
  "IW{1,1}(19,:)'" : Constant  Value=[-0.0980450133267183610019657180600916035473346710205078125;-0.1312971944880636787633676476616528816521167755126953125;0.39294263311544852523837789703975431621074676513671875;-0.41124084417166584248803928858251310884952545166015625;0.262763920808531115103079400796559639275074005126953125;-0.88060866943884053004154566224315203726291656494140625;-0.85165929259127570727372358305728994309902191162109375;0.48336938542803853380291911889798939228057861328125]
      mask Display: e = 0.06;c1 = [120 150 230]/255;c2 = ([120 150 230]+0)/383;c3 = ([120 150 230]+128)/383;patch([0 1 1 0],[0 0 1 1],c1);patch([0 1 1 1-e 1-e 0+e],[0 0 1 1-e 0+e 0+e],c2);patch([0 0 1 1-e 0+e 0+e],[0 1 1 1-e 1-e 0+e],c3);plot([0 1 1 0 0],[0 0 1 1 0]);disp('Weights');
  "IW{1,1}(2,:)'" : Constant  Value=[-0.0002054311605086852330660784904381443993770517408847808837890625;-0.008493020638395909482909473808831535279750823974609375;-0.1013652639524386389613397341236122883856296539306640625;-0.0288894493846899684530438179308475810103118419647216796875;-1.2951744345640339162173404474742710590362548828125;-0.213669199678342025539024007230182178318500518798828125;1.46815248202260750787218057666905224323272705078125;1.354131895636293325679844201658852398395538330078125]
      mask Display: e = 0.06;c1 = [120 150 230]/255;c2 = ([120 150 230]+0)/383;c3 = ([120 150 230]+128)/383;patch([0 1 1 0],[0 0 1 1],c1);patch([0 1 1 1-e 1-e 0+e],[0 0 1 1-e 0+e 0+e],c2);patch([0 0 1 1-e 0+e 0+e],[0 1 1 1-e 1-e 0+e],c3);plot([0 1 1 0 0],[0 0 1 1 0]);disp('Weights');
  "IW{1,1}(20,:)'" : Constant  Value=[-0.39123095173069588614822578165330924093723297119140625;0.29743779210468834772740365224308334290981292724609375;-0.0275588411168332415857040729179061600007116794586181640625;-0.419880350563146986786478009889833629131317138671875;-0.615084781617870834935501989093609154224395751953125;0.09547250073506298451153639916810789145529270172119140625;1.09093140752721939890079738688655197620391845703125;0.840598493940383217903900003875605762004852294921875]
      mask Display: e = 0.06;c1 = [120 150 230]/255;c2 = ([120 150 230]+0)/383;c3 = ([120 150 230]+128)/383;patch([0 1 1 0],[0 0 1 1],c1);patch([0 1 1 1-e 1-e 0+e],[0 0 1 1-e 0+e 0+e],c2);patch([0 0 1 1-e 0+e 0+e],[0 1 1 1-e 1-e 0+e],c3);plot([0 1 1 0 0],[0 0 1 1 0]);disp('Weights');
  "IW{1,1}(3,:)'" : Constant  Value=[-0.2379011132694721364355672221790882758796215057373046875;0.228186974793161689856191287617548368871212005615234375;0.6931252694762155552865579011267982423305511474609375;0.8036057418458846246522853107308037579059600830078125;0.17843631735289100515018390069599263370037078857421875;-1.2457006116102415926860658146324567496776580810546875;-0.58716353248966368649774949517450295388698577880859375;-0.3831546588055108060189013485796749591827392578125]
      mask Display: e = 0.06;c1 = [120 150 230]/255;c2 = ([120 150 230]+0)/383;c3 = ([120 150 230]+128)/383;patch([0 1 1 0],[0 0 1 1],c1);patch([0 1 1 1-e 1-e 0+e],[0 0 1 1-e 0+e 0+e],c2);patch([0 0 1 1-e 0+e 0+e],[0 1 1 1-e 1-e 0+e],c3);plot([0 1 1 0 0],[0 0 1 1 0]);disp('Weights');
  "IW{1,1}(4,:)'" : Constant  Value=[0.0251197275992513548159568159690024913288652896881103515625;-0.03969457888013601387644513351915520615875720977783203125;0.2873518497159324169842875562608242034912109375;-0.03748538218542372957298169922069064341485500335693359375;0.80783229761712271876916702240123413503170013427734375;0.704192697723136529219800650025717914104461669921875;-1.0818965792260828440163322738953866064548492431640625;-1.1181826473672813460069619395653717219829559326171875]
      mask Display: e = 0.06;c1 = [120 150 230]/255;c2 = ([120 150 230]+0)/383;c3 = ([120 150 230]+128)/383;patch([0 1 1 0],[0 0 1 1],c1);patch([0 1 1 1-e 1-e 0+e],[0 0 1 1-e 0+e 0+e],c2);patch([0 0 1 1-e 0+e 0+e],[0 1 1 1-e 1-e 0+e],c3);plot([0 1 1 0 0],[0 0 1 1 0]);disp('Weights');
  "IW{1,1}(5,:)'" : Constant  Value=[-0.041768040591042283893319364551643957383930683135986328125;0.038218305831577432940537875083464314229786396026611328125;0.64242665473583604462959328884608112275600433349609375;1.0989998379862704336318302011932246387004852294921875;-0.407168576964892281466745771467685699462890625;1.3737044161391682717265894098090939223766326904296875;0.208672052560637644180729921572492457926273345947265625;-0.255087655492435005921691981711774133145809173583984375]
      mask Display: e = 0.06;c1 = [120 150 230]/255;c2 = ([120 150 230]+0)/383;c3 = ([120 150 230]+128)/383;patch([0 1 1 0],[0 0 1 1],c1);patch([0 1 1 1-e 1-e 0+e],[0 0 1 1-e 0+e 0+e],c2);patch([0 0 1 1-e 0+e 0+e],[0 1 1 1-e 1-e 0+e],c3);plot([0 1 1 0 0],[0 0 1 1 0]);disp('Weights');
  "IW{1,1}(6,:)'" : Constant  Value=[0.033006669381857943468272509335292852483689785003662109375;-0.1056122386414183045300063668037182651460170745849609375;0.2276256265538296741368640141445212066173553466796875;0.55126615490331232205534206514130346477031707763671875;0.403042148616312101427894276639563031494617462158203125;-0.705631924844520863615571215632371604442596435546875;-0.89528063381783606899944061296992003917694091796875;0.34863383801820102547708302154205739498138427734375]
      mask Display: e = 0.06;c1 = [120 150 230]/255;c2 = ([120 150 230]+0)/383;c3 = ([120 150 230]+128)/383;patch([0 1 1 0],[0 0 1 1],c1);patch([0 1 1 1-e 1-e 0+e],[0 0 1 1-e 0+e 0+e],c2);patch([0 0 1 1-e 0+e 0+e],[0 1 1 1-e 1-e 0+e],c3);plot([0 1 1 0 0],[0 0 1 1 0]);disp('Weights');
  "IW{1,1}(7,:)'" : Constant  Value=[-0.0271822433727387409441167420709462021477520465850830078125;0.004464420990478035720927518781309117912314832210540771484375;0.0260878196663470972305187700612805201672017574310302734375;0.020967305039616114525902190734996111132204532623291015625;-0.1601202478582996746592215231430600397288799285888671875;-0.8928253539156403295606878600665368139743804931640625;-0.038382124628219056738931413974569295533001422882080078125;-1.1373422376243380593763276920071803033351898193359375]
      mask Display: e = 0.06;c1 = [120 150 230]/255;c2 = ([120 150 230]+0)/383;c3 = ([120 150 230]+128)/383;patch([0 1 1 0],[0 0 1 1],c1);patch([0 1 1 1-e 1-e 0+e],[0 0 1 1-e 0+e 0+e],c2);patch([0 0 1 1-e 0+e 0+e],[0 1 1 1-e 1-e 0+e],c3);plot([0 1 1 0 0],[0 0 1 1 0]);disp('Weights');
  "IW{1,1}(8,:)'" : Constant  Value=[-0.0008903569142505556033295732731858151964843273162841796875;-0.003561944625287568298721563309072735137306153774261474609375;0.036619504766960388197905018614619621075689792633056640625;-0.05389776702857436430083026834836346097290515899658203125;-0.384328242703213474040779829010716639459133148193359375;0.8598302102658286205638660248951055109500885009765625;0.631580292214194205513422275544144213199615478515625;-1.589124006465480132277434677234850823879241943359375]
      mask Display: e = 0.06;c1 = [120 150 230]/255;c2 = ([120 150 230]+0)/383;c3 = ([120 150 230]+128)/383;patch([0 1 1 0],[0 0 1 1],c1);patch([0 1 1 1-e 1-e 0+e],[0 0 1 1-e 0+e 0+e],c2);patch([0 0 1 1-e 0+e 0+e],[0 1 1 1-e 1-e 0+e],c3);plot([0 1 1 0 0],[0 0 1 1 0]);disp('Weights');
  "IW{1,1}(9,:)'" : Constant  Value=[-0.049854519928796685312999414918522234074771404266357421875;0.10068300480426829734970084473388851620256900787353515625;-0.1894841333097706803645365880583995021879673004150390625;-0.05050382235759136306807448590916465036571025848388671875;-0.307014760978943479496905410996987484395503997802734375;-0.05322280824341962812695783213712275028228759765625;-0.475975482587448650573236363925389014184474945068359375;0.26615814025558048871999972107005305588245391845703125]
      mask Display: e = 0.06;c1 = [120 150 230]/255;c2 = ([120 150 230]+0)/383;c3 = ([120 150 230]+128)/383;patch([0 1 1 0],[0 0 1 1],c1);patch([0 1 1 1-e 1-e 0+e],[0 0 1 1-e 0+e 0+e],c2);patch([0 0 1 1-e 0+e 0+e],[0 1 1 1-e 1-e 0+e],c3);plot([0 1 1 0 0],[0 0 1 1 0]);disp('Weights');
  Mux : Mux  Inputs=20
      mask Display: e = 0.06;c1 = [120 150 230]/255;c2 = ([120 150 230]+0)/383;c3 = ([120 150 230]+128)/383;patch([0 1 1 0],[0 0 1 1],c1);patch([0 1 1 1-e 1-e 0+e],[0 0 1 1-e 0+e 0+e],c2);patch([0 0 1 1-e 0+e 0+e],[0 1 1 1-e 1-e 0+e],c3);plot([0 1 1 0 0],[0 0 1 1 0]);disp('Mux');
  dotprod{1..20} (20 alike) : neural/Weight Functions/dotprod
  "iz{1,1}" : Outport
      mask Display: e = 0.06;c1 = [120 230 180]/255;c2 = ([120 230 180]+0)/(256+128);c3 = ([120 230 180]+128)/(256+128);patch([0 1 1 0],[0 0 1 1],c1);patch([0 1 1 1-e 1-e 0+e],[0 0 1 1-e 0+e 0+e],c2);patch([0 0 1 1-e 0+e 0+e],[0 1 1 1-e 1-e 0+e],c3);plot([0 1 1 0 0],[0 0 1 1 0]);
  wires:
  "IW{1,1}(1,:)'"/1 -> dotprod1/1
  "pd{1,1}"/1 -> dotprod1/2, dotprod2/2, dotprod3/2, dotprod4/2, dotprod5/2, dotprod6/2, dotprod7/2, dotprod8/2, dotprod9/2, dotprod10/2, dotprod11/2, dotprod12/2, dotprod13/2, dotprod14/2, dotprod15/2, dotprod16/2, dotprod17/2, dotprod18/2, dotprod19/2, dotprod20/2
  dotprod1/1 -> Mux/1
  "IW{1,1}(2,:)'"/1 -> dotprod2/1
  dotprod2/1 -> Mux/2
  "IW{1,1}(3,:)'"/1 -> dotprod3/1
  dotprod3/1 -> Mux/3
  "IW{1,1}(4,:)'"/1 -> dotprod4/1
  dotprod4/1 -> Mux/4
  "IW{1,1}(5,:)'"/1 -> dotprod5/1
  dotprod5/1 -> Mux/5
  "IW{1,1}(6,:)'"/1 -> dotprod6/1
  dotprod6/1 -> Mux/6
  "IW{1,1}(7,:)'"/1 -> dotprod7/1
  dotprod7/1 -> Mux/7
  "IW{1,1}(8,:)'"/1 -> dotprod8/1
  dotprod8/1 -> Mux/8
  "IW{1,1}(9,:)'"/1 -> dotprod9/1
  dotprod9/1 -> Mux/9
  "IW{1,1}(10,:)'"/1 -> dotprod10/1
  dotprod10/1 -> Mux/10
  "IW{1,1}(11,:)'"/1 -> dotprod11/1
  dotprod11/1 -> Mux/11
  "IW{1,1}(12,:)'"/1 -> dotprod12/1
  dotprod12/1 -> Mux/12
  "IW{1,1}(13,:)'"/1 -> dotprod13/1
  dotprod13/1 -> Mux/13
  "IW{1,1}(14,:)'"/1 -> dotprod14/1
  dotprod14/1 -> Mux/14
  "IW{1,1}(15,:)'"/1 -> dotprod15/1
  dotprod15/1 -> Mux/15
  "IW{1,1}(16,:)'"/1 -> dotprod16/1
  dotprod16/1 -> Mux/16
  "IW{1,1}(17,:)'"/1 -> dotprod17/1
  dotprod17/1 -> Mux/17
  "IW{1,1}(18,:)'"/1 -> dotprod18/1
  dotprod18/1 -> Mux/18
  "IW{1,1}(19,:)'"/1 -> dotprod19/1
  dotprod19/1 -> Mux/19
  "IW{1,1}(20,:)'"/1 -> dotprod20/1
  dotprod20/1 -> Mux/20
  Mux/1 -> "iz{1,1}"/1

== system test_direct/Function Fitting Neural Network4/Layer 2/Delays 1 ==
  "p{2}" : Inport  PortDimensions=20
      mask Display: e = 0.06;c1 = [120 230 180]/255;c2 = ([120 230 180]+0)/(256+128);c3 = ([120 230 180]+128)/(256+128);patch([0 1 1 0],[0 0 1 1],c1);patch([0 1 1 1-e 1-e 0+e],[0 0 1 1-e 0+e 0+e],c2);patch([0 0 1 1-e 0+e 0+e],[0 1 1 1-e 1-e 0+e],c3);plot([0 1 1 0 0],[0 0 1 1 0]);
  mux : Mux  Inputs=1
      mask Display: e = 0.06;c1 = [120 150 230]/255;c2 = ([120 150 230]+0)/383;c3 = ([120 150 230]+128)/383;patch([0 1 1 0],[0 0 1 1],c1);patch([0 1 1 1-e 1-e 0+e],[0 0 1 1-e 0+e 0+e],c2);patch([0 0 1 1-e 0+e 0+e],[0 1 1 1-e 1-e 0+e],c3);plot([0 1 1 0 0],[0 0 1 1 0]);disp('Mux')
  "pd{2,1}" : Outport
      mask Display: e = 0.06;c1 = [120 230 180]/255;c2 = ([120 230 180]+0)/(256+128);c3 = ([120 230 180]+128)/(256+128);patch([0 1 1 0],[0 0 1 1],c1);patch([0 1 1 1-e 1-e 0+e],[0 0 1 1-e 0+e 0+e],c2);patch([0 0 1 1-e 0+e 0+e],[0 1 1 1-e 1-e 0+e],c3);plot([0 1 1 0 0],[0 0 1 1 0]);
  wires:
  "p{2}"/1 -> mux/1
  mux/1 -> "pd{2,1}"/1
